simulink model "dcMotorSim"  (Simulink 9.0)
settings: Solver=VariableStepAuto  StartTime=0.0  StopTime=10  RelTol=1e-3
values from neighbouring files (symbols this model uses):
  J = 0.181    [dcMotorPar.m]
  kb = 36.9e-3    (= 0.0369)    [dcMotorPar.m]
  kf = 0.1    [dcMotorPar.m]
  km = 20    [dcMotorPar.m]
  L = 0.463e-3    (= 0.000463)    [dcMotorPar.m]
  R = 0.608    [dcMotorPar.m]
settings Model: Creator=chsl  LastModifiedBy=chsl
settings DataIOCC: SaveFormat=Dataset
settings OptimizationCC: LifeSpan=auto
settings DebuggingCC: UnderspecifiedInitializationDetection=Simplified  MergeDetectMultiDrivingBlocksExec=error  SFUnexpectedBacktrackingDiag=error  SFNoUnconditionalDefaultTransitionDiag=error  SFExecutionAtInitializationDiag=warning
settings HardwareCC: ProdBitPerPointer=64  ProdBitPerSizeT=64  ProdBitPerPtrDiffT=64  ProdLargestAtomicFloat=Float  ProdIntDivRoundTo=Zero  ProdEndianess=LittleEndian  ProdWordSize=64  ProdHWDeviceType=Intel->x86-64 (Windows64)
settings ModelReferenceCC: PropagateSignalLabelsOutOfModel=on
settings CodeAppCC: StateflowObjectComments=off
settings GRTTargetCC: TargetLangStandard=C99 (ISO)
settings ConfigComp: CovMetricSettings=dwe  CovHtmlReporting=off  CovSaveCumulativeToWorkspaceVar=off  CovSaveSingleToWorkspaceVar=off  CovExternalEMLEnable=on

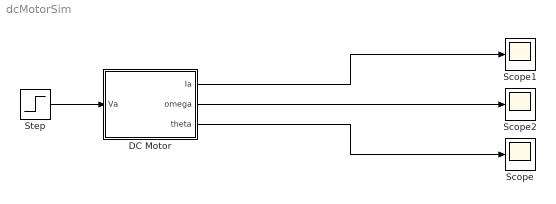
== system dcMotorSim ==
  DC Motor : Subsystem
  Scope : Scope
  Scope1 : Scope
  Scope2 : Scope
  Step : Step  SampleTime=0
  wires:
  DC Motor/3(theta) -> Scope/1
  DC Motor/1(Ia) -> Scope1/1
  DC Motor/2(omega) -> Scope2/1
  Step/1 -> DC Motor/1(Va)

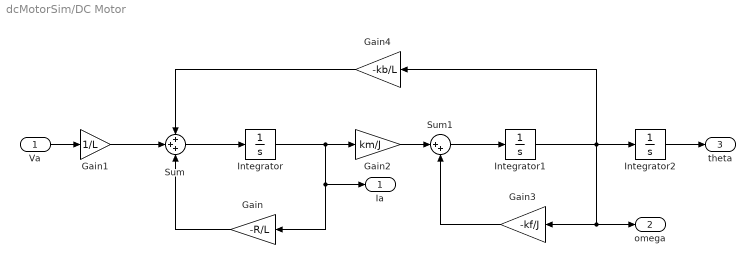
== system dcMotorSim/DC Motor ==
  Va : Inport
  Gain : Gain  Gain=-R/L
  Gain1 : Gain  Gain=1/L
  Gain2 : Gain  Gain=km/J
  Gain3 : Gain  Gain=-kf/J
  Gain4 : Gain  Gain=-kb/L
  Integrator : Integrator
  Integrator1 : Integrator
  Integrator2 : Integrator
  Sum : Sum  Inputs=+++
  Sum1 : Sum  Inputs=|++
  Ia : Outport
  omega : Outport  Port=2
  theta : Outport  Port=3
  wires:
  Gain2/1 -> Sum1/1
  Integrator1/1 -> Gain4/1, omega/1, Gain3/1, Integrator2/1
  Integrator/1 -> Ia/1, Gain/1, Gain2/1
  Sum/1 -> Integrator/1
  Va/1 -> Gain1/1
  Gain1/1 -> Sum/2
  Gain3/1 -> Sum1/2
  Integrator2/1 -> theta/1
  Gain4/1 -> Sum/1
  Sum1/1 -> Integrator1/1
  Gain/1 -> Sum/3
